simulink model "QUESTION4_4"  (R2021a)
settings: Solver=VariableStepAuto  StartTime=0.0  StopTime=10.0  RelTol=1e-3
settings Model: Creator=user  LastModifiedBy=user

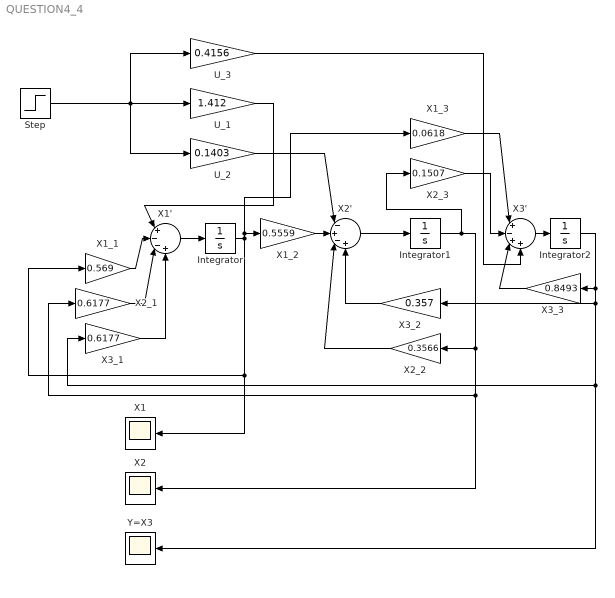
== system QUESTION4_4 ==
  Integrator : Integrator
  Integrator1 : Integrator
  Integrator2 : Integrator
  Step : Step  SampleTime=0
  U_1 : Gain  Gain=1.412
  U_2 : Gain  Gain=0.1403
  U_3 : Gain  Gain=0.4156
  X1 : Scope
  X1' : Sum  Inputs=|+--+
  X1_1 : Gain  Gain=0.569
  X1_2 : Gain  Gain=0.5559
  X1_3 : Gain  Gain=0.0618
  X2 : Scope
  X2' : Sum  Inputs=|-+-+
  X2_1 : Gain  Gain=0.6177
  X2_2 : Gain  Gain=0.3566
  X2_3 : Gain  Gain=0.1507
  X3' : Sum  Inputs=|+-++
  X3_1 : Gain  Gain=0.6177
  X3_2 : Gain  Gain=0.357
  X3_3 : Gain  Gain=0.8493
  Y=X3 : Scope
  wires:
  Integrator1/1 -> X2_3/1, X2_2/1, X2_1/1, X2/1
  X3'/1 -> Integrator2/1
  X1'/1 -> Integrator/1
  Integrator2/1 -> X3_3/1, X3_1/1, Y=X3/1, X3_2/1
  X2'/1 -> Integrator1/1
  Step/1 -> U_3/1, U_1/1, U_2/1
  U_2/1 -> X2'/1
  X3_2/1 -> X2'/4
  X2_2/1 -> X2'/3
  X1_2/1 -> X2'/2
  X2_3/1 -> X3'/2
  Integrator/1 -> X1_3/1, X1_2/1, X1_1/1, X1/1
  X1_3/1 -> X3'/1
  U_1/1 -> X1'/1
  X3_1/1 -> X1'/4
  X2_1/1 -> X1'/3
  X1_1/1 -> X1'/2
  X3_3/1 -> X3'/3
  U_3/1 -> X3'/4
